simulink model "ZN_cl_saturation_weighted_s"  (R2021b)
settings: Solver=VariableStepAuto  StartTime=0.0  StopTime=20  RelTol=1e-3
settings Model: Creator=nima8  LastModifiedBy=nima8

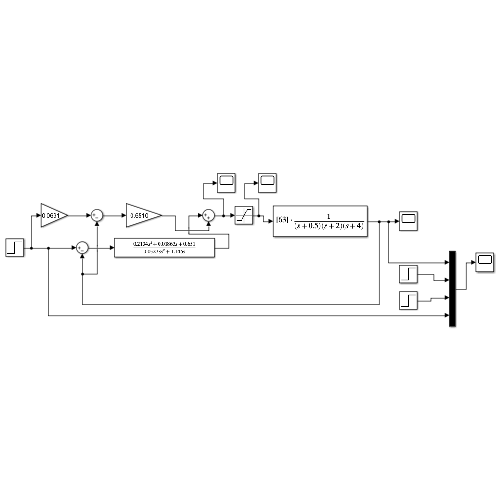
[thumbnail: Simulink's stored preview of the top-level diagram]
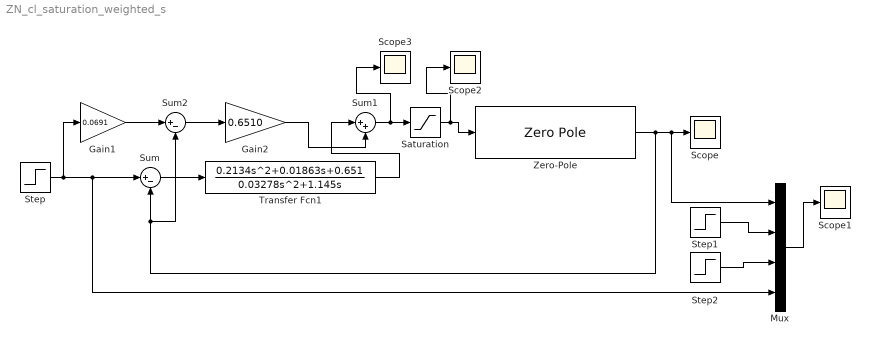
== system ZN_cl_saturation_weighted_s ==
  Gain1 : Gain  Gain=0.0691
  Gain2 : Gain  Gain=0.6510
  Mux : Mux
  Saturation : Saturate  UpperLimit=4.55  LowerLimit=0.1
  Scope{,1..3} (4 alike) : Scope
  Step : Step  Time=0  SampleTime=0
  Step1 : Step  Time=0  After=0.98  SampleTime=0
  Step2 : Step  Time=0  After=1.02  SampleTime=0
  Sum : Sum  Inputs=|+-
  Sum1 : Sum  Inputs=|++
  Sum2 : Sum  Inputs=|+-
  Transfer Fcn1 : TransferFcn  Numerator=[0.2134 0.01863 0.651]  Denominator=[0.03278 1.145 0]
  Zero-Pole : ZeroPole  Zeros=[]  Poles=[-0.5 -2 -4]  Gain=[63]
  wires:
  Mux/1 -> Scope1/1
  Transfer Fcn1/1 -> Sum1/1
  Zero-Pole/1 -> Mux/1, Scope/1, Sum2/2, Sum/2
  Step2/1 -> Mux/3
  Step/1 -> Gain1/1, Mux/4, Sum/1
  Gain2/1 -> Sum1/2
  Sum/1 -> Transfer Fcn1/1
  Gain1/1 -> Sum2/1
  Step1/1 -> Mux/2
  Sum2/1 -> Gain2/1
  Saturation/1 -> Scope2/1, Zero-Pole/1
  Sum1/1 -> Scope3/1, Saturation/1
